simulink model "main"  (R2016b)
settings: Solver=FixedStepAuto  StartTime=0.0  StopTime=inf  FixedStep=Ts  MaxStep=0.2  RelTol=1e-2
undefined symbols (not defined in the file): checks, datetime, decyear, delta_e, deltae_degrees, deltafl_degrees, deltafr_degrees, deltar_degrees, deltat_1, deltat_2, deltat_3, deltat_4, deltat_5, Earth, F, ft, groundReaction, initialValues, juliandate, LD, leapyear, Light, m, MIL, Newton, Raphson, s, sigbuilder_block, Ts, WGS84
libraries: simulink x68, aerolibutil x17, aerolibtransform2 x15, simulink_extras x13, aerolibasang x5, aerolib6dofsys x5, aerolib6dof2 x4, aerolibwind2 x3, aerolibbdyn x3, vrlib x3, aerolibconvert2 x3, aerolibactuator x2
(part 8 of 10)

== system main/LIBIS Plant/Propulsion/Variant_Motor_5 ==
  note: 1) Add Subsystem or Model blocks as valid variant choices.
      | 2) You cannot connect blocks at this level. At simulation, connectivity is automatically
      | determined, based on the active variant and port name matching.
  Vbattery : Inport
  Throttle : Inport  Port=2
  envData : Inport  Port=3
  plantData : Inport  Port=4
  mappedMotor_5 : Subsystem  VariantControl=mappedMotors==1
  noMappedMotor_5 : Subsystem  VariantControl=mappedMotors~=1
  Im : Outport
  Thrust : Outport  Port=2
  Thrust_moment : Outport  Port=3

== system main/LIBIS Plant/Subsystem/calc alpha_dot ==
  q : Inport
  alpha,beta : Inport  Port=2
  Ab : Inport  Port=3
  Vw : Inport  Port=4
  Direction Cosine Matrix Body to Wind : aerolibtransform2/Direction Cosine Matrix Body to Wind
  Product1 : Product  Multiplication=Matrix(*)  SaturateOnIntegerOverflow=on  InputSameDT=on  OutDataTypeStr=Inherit: Same as first input
  Product2 : Product  Inputs=*/  SaturateOnIntegerOverflow=on  InputSameDT=on  OutDataTypeStr=Inherit: Same as first input
  Selector2 : Selector  IndexMode=Zero-based  InputPortWidth=3  IndexOptions=Index vector (dialog)  Indices=2  OutputSizes=1
  Selector3 : Selector  IndexMode=Zero-based  InputPortWidth=3  IndexOptions=Index vector (dialog)  Indices=0  OutputSizes=1
  Sum : Sum  Inputs=++|
  Transpose1 : Math  Operator=transpose  SaturateOnIntegerOverflow=on
  alpha_dot : Outport
  wires:
  Direction Cosine Matrix Body to Wind/1 -> Transpose1/1
  Transpose1/1 -> Product1/1
  Product1/1 -> Selector2/1
  Selector2/1 -> Product2/1
  Selector3/1 -> Product2/2
  Product2/1 -> Sum/2
  alpha,beta/1 -> Direction Cosine Matrix Body to Wind/1
  q/1 -> Sum/1
  Sum/1 -> alpha_dot/1
  Ab/1 -> Product1/2
  Vw/1 -> Selector3/1

== system main/LIBIS Plant/alpha_dot, beta_dot/Subsystem ==
  beta : Inport  Unit=rad
  alpha : Inport  Port=2  Unit=rad
  V_body : Inport  Port=3  Unit=meter/s
  Omega_body : Inport  Port=4  Unit=rad/s
  Accel_body : Inport  Port=5  Unit=m/s^2
  Constant11 : Constant  Value=0
  Direction Cosine Matrix Body to Wind : aerolibtransform2/Direction Cosine Matrix Body to Wind
  Mux4 : Mux  Inputs=2
  Product1 : Product  Multiplication=Matrix(*)  SaturateOnIntegerOverflow=on  InputSameDT=on  OutDataTypeStr=Inherit: Same as first input
  Selector : Selector  InputPortWidth=3  IndexOptions=Index vector (dialog)  Indices=[2]  OutputSizes=1
  calc alpha_dot : Subsystem
  alpha_dot : Outport  Unit=rad/s
  beta_dot : Outport  Port=2
  wires:
  Direction Cosine Matrix Body to Wind/1 -> Product1/1
  Product1/1 -> calc alpha_dot/4(Vw)
  Mux4/1 -> Direction Cosine Matrix Body to Wind/1, calc alpha_dot/2(alpha,beta)
  Constant11/1 -> beta_dot/1  "beta_dot"
  alpha/1 -> Mux4/1
  Omega_body/1 -> Selector/1
  V_body/1 -> Product1/2
  Accel_body/1 -> calc alpha_dot/3(Ab)
  beta/1 -> Mux4/2
  calc alpha_dot/1(alpha_dot) -> alpha_dot/1
  Selector/1 -> calc alpha_dot/1(q)  "q"

== system main/Sensors/Feedthrough Sensors/CPU ==
  States : Inport  OutDataTypeStr=Bus: plantDataBus
  Bus Selector : BusSelector  OutputSignals=CG,remainingCapacity
  CGMeas : Outport
  remainingCapacityMeas : Outport  Port=2
  wires:
  States/1 -> Bus Selector/1  "plantData"
  Bus Selector/1 -> CGMeas/1  "<CG>"
  Bus Selector/2 -> remainingCapacityMeas/1  "<remainingCapacity>"

== system main/Sensors/Feedthrough Sensors/GPS ==
  States : Inport  OutDataTypeStr=Bus: plantDataBus
  Bus Creator : BusCreator  Inputs='LatitudeMeas_deg','LongitudeMeas_deg','AltitudeMeas_m'  OutDataTypeStr=Bus: LLAMeasBus  NonVirtualBus=on
  Bus Selector : BusSelector  OutputSignals=LLA.Latitude_deg,LLA.Longitude_deg,LLA.Altitude_m
  Constant13 : Constant  Value=initialValues.href
  Derivative : Derivative
  LLA to Flat Earth : aerolibtransform2/LLA to Flat Earth  units=Metric (MKS)  ptype=Earth (WGS84)  F=1/298.257223563  R=6378137  LL0=initialValues.LatLong0  psi=0
  Mux2 : Mux  Inputs=2
  Signal Specification : SignalSpecification
  Signal Specification1 : SignalSpecification
  Signal Specification2 : SignalSpecification
  LLAMeas : Outport  OutDataTypeStr=Bus: LLAMeasBus
  X_nedMeas : Outport  Port=2
  VearthMeas : Outport  Port=3
  wires:
  Bus Creator/1 -> LLAMeas/1  "LLAMeas"
  Bus Selector/1 -> Signal Specification/1  "<Latitude_deg>"
  Bus Selector/3 -> Signal Specification2/1  "<Altitude_m>"
  Bus Selector/2 -> Signal Specification1/1  "<Longitude_deg>"
  Signal Specification/1 -> Mux2/1, Bus Creator/1  "LatitudeMeas_deg"
  Signal Specification1/1 -> Mux2/2, Bus Creator/2  "LongitudeMeas_deg"
  Signal Specification2/1 -> LLA to Flat Earth/2, Bus Creator/3  "AltitudeMeas_m"
  States/1 -> Bus Selector/1  "plantData"
  Constant13/1 -> LLA to Flat Earth/3
  Mux2/1 -> LLA to Flat Earth/1
  LLA to Flat Earth/1 -> Derivative/1, X_nedMeas/1  "X_NedMeas"
  Derivative/1 -> VearthMeas/1

== system main/Sensors/Feedthrough Sensors/IMU ==
  States : Inport  OutDataTypeStr=Bus: plantDataBus
  Environment : Inport  Port=2  OutDataTypeStr=Bus: envDataBus
  Bus Creator : BusCreator  Inputs='pMeas','qMeas','rMeas'  OutDataTypeStr=Bus: OmegaMeasBus  NonVirtualBus=on
  Bus Selector : BusSelector  OutputSignals=Accel_body,Omega_body.p,Omega_body.q,Omega_body.r,dOmega_body,CG,DCM_body_earth
  Bus Selector1 : BusSelector  OutputSignals=Gravity_ned
  Calculate DCM & Euler Angles : Subsystem
  Demux : Demux  Outputs=3
  Mux : Mux  Inputs=3
  Mux1 : Mux  Inputs=3
  Product : Product  Multiplication=Matrix(*)
  Three-axis Inertial Measurement Unit : aerolibnav/Three-axis Inertial Measurement Unit  units=Metric (MKS)  imu=[0 0 0]  i_Ts=0  dtype_a=off  w_a=190  z_a=1  a_sf_cc=[1 0 0; 0 1 0; 0 0 1]  a_bias=[0 0 0]  a_sat="[-inf  -inf  -inf  inf inf inf]"  dtype_g=off  w_g=190  z_g=1  g_sf_cc=[1 0 0; 0 1 0; 0 0 1]  g_bias=[0 0 0]  g_sens=[0 0 0]  g_sat="[-inf  -inf  -inf  inf inf inf]"  i_rand=off  i_seeds=[23093 23094 23095 23096 23097 23098]  i_pow=[0.001 0.001 0.001 0.0001 0.0001 0.0001]
  AccelMeas_body : Outport
  OmegaMeas_body : Outport  Port=2  OutDataTypeStr=Bus: OmegaMeasBus
  DCMMeas_body_earth : Outport  Port=3
  EulerMeas : Outport  Port=4
  wires:
  Demux/1 -> Mux/1, Bus Creator/1  "pMeas"
  Demux/2 -> Mux/2, Bus Creator/2  "qMeas"
  Demux/3 -> Mux/3, Bus Creator/3  "rMeas"
  Calculate DCM & Euler Angles/1(DCMMeas) -> DCMMeas_body_earth/1
  Calculate DCM & Euler Angles/2(EulerMeas) -> EulerMeas/1
  Mux/1 -> Calculate DCM & Euler Angles/1("p q r ")
  Three-axis Inertial Measurement Unit/1 -> AccelMeas_body/1
  Bus Creator/1 -> OmegaMeas_body/1
  Three-axis Inertial Measurement Unit/2 -> Demux/1
  States/1 -> Bus Selector/1  "plantData"
  Bus Selector/4 -> Mux1/3  "<r>"
  Bus Selector/3 -> Mux1/2  "<q>"
  Bus Selector/2 -> Mux1/1  "<p>"
  Environment/1 -> Bus Selector1/1  "Environment"
  Bus Selector1/1 -> Product/2  "<Gravity_ned>"
  Mux1/1 -> Three-axis Inertial Measurement Unit/2  "Omega_body"
  Bus Selector/1 -> Three-axis Inertial Measurement Unit/1  "<Accel_body>"
  Bus Selector/6 -> Three-axis Inertial Measurement Unit/4  "<CG>"
  Bus Selector/5 -> Three-axis Inertial Measurement Unit/3  "<dOmega_body>"
  Bus Selector/7 -> Product/1  "<DCM_body_earth>"
  Product/1 -> Three-axis Inertial Measurement Unit/5

== system main/Sensors/Feedthrough Sensors/Pitot ==
  States : Inport  OutDataTypeStr=Bus: plantDataBus
  Environment : Inport  Port=2  OutDataTypeStr=Bus: envDataBus
  Bus Selector : BusSelector  OutputSignals=V_body
  Bus Selector1 : BusSelector  OutputSignals=windVelocity
  Sum : Sum  Inputs=|+-
  VaeroMeas_body : Outport
  wires:
  Bus Selector/1 -> Sum/1  "<V_body>"
  States/1 -> Bus Selector/1  "plantData"
  Environment/1 -> Bus Selector1/1
  Bus Selector1/1 -> Sum/2  "<windVelocity>"
  Sum/1 -> VaeroMeas_body/1  "VaeroMeas_body"

== system main/Sensors/Feedthrough Sensors/Veleta ==
  States : Inport  OutDataTypeStr=Bus: plantDataBus
  Bus Selector : BusSelector  OutputSignals=alpha,beta
  alphaMeas : Outport
  betaMeas : Outport  Port=2
  wires:
  States/1 -> Bus Selector/1  "plantData"
  Bus Selector/1 -> alphaMeas/1  "<alpha>"
  Bus Selector/2 -> betaMeas/1  "<beta>"

== system main/Sensors/Noisy Sensors/CPU (Feedthough) ==
  States : Inport  OutDataTypeStr=Bus: plantDataBus
  Bus Selector : BusSelector  OutputSignals=CG,remainingCapacity
  CGMeas : Outport
  remainingCapacityMeas : Outport  Port=2
  wires:
  States/1 -> Bus Selector/1  "plantData"
  Bus Selector/1 -> CGMeas/1  "<CG>"
  Bus Selector/2 -> remainingCapacityMeas/1  "<remainingCapacity>"

== system main/Sensors/Noisy Sensors/GPS (Feedthough) ==
  States : Inport  OutDataTypeStr=Bus: plantDataBus
  Bus Creator : BusCreator  Inputs='LatitudeMeas_deg','LongitudeMeas_deg','AltitudeMeas_m'  OutDataTypeStr=Bus: LLAMeasBus  NonVirtualBus=on
  Bus Selector : BusSelector  OutputSignals=LLA.Latitude_deg,LLA.Longitude_deg,LLA.Altitude_m
  Constant13 : Constant  Value=initialValues.href
  Derivative : Derivative
  LLA to Flat Earth : aerolibtransform2/LLA to Flat Earth  units=Metric (MKS)  ptype=Earth (WGS84)  F=1/298.257223563  R=6378137  LL0=initialValues.LatLong0  psi=0
  Mux2 : Mux  Inputs=2
  Signal Specification : SignalSpecification
  Signal Specification1 : SignalSpecification
  Signal Specification2 : SignalSpecification
  LLAMeas : Outport  OutDataTypeStr=Bus: LLAMeasBus
  X_nedMeas : Outport  Port=2
  VearthMeas : Outport  Port=3
  wires:
  Bus Creator/1 -> LLAMeas/1  "LLAMeas"
  Bus Selector/1 -> Signal Specification/1  "<Latitude_deg>"
  Bus Selector/3 -> Signal Specification2/1  "<Altitude_m>"
  Bus Selector/2 -> Signal Specification1/1  "<Longitude_deg>"
  Signal Specification/1 -> Mux2/1, Bus Creator/1  "LatitudeMeas_deg"
  Signal Specification1/1 -> Mux2/2, Bus Creator/2  "LongitudeMeas_deg"
  Signal Specification2/1 -> LLA to Flat Earth/2, Bus Creator/3  "AltitudeMeas_m"
  States/1 -> Bus Selector/1  "plantData"
  Constant13/1 -> LLA to Flat Earth/3
  Mux2/1 -> LLA to Flat Earth/1
  LLA to Flat Earth/1 -> Derivative/1, X_nedMeas/1  "X_NedMeas"
  Derivative/1 -> VearthMeas/1

== system main/Sensors/Noisy Sensors/IMU ==
  States : Inport  OutDataTypeStr=Bus: plantDataBus
  Environment : Inport  Port=2  OutDataTypeStr=Bus: envDataBus
  Bus Creator : BusCreator  Inputs='pMeas','qMeas','rMeas'  OutDataTypeStr=Bus: OmegaMeasBus  NonVirtualBus=on
  Bus Selector : BusSelector  OutputSignals=Accel_body,Omega_body.p,Omega_body.q,Omega_body.r,dOmega_body,CG,DCM_body_earth
  Bus Selector1 : BusSelector  OutputSignals=Gravity_ned
  Calculate DCM & Euler Angles : Subsystem
  Demux : Demux  Outputs=3
  Mux : Mux  Inputs=3
  Mux1 : Mux  Inputs=3
  Product : Product  Multiplication=Matrix(*)
  Three-axis Inertial Measurement Unit : aerolibnav/Three-axis Inertial Measurement Unit  units=Metric (MKS)  imu=[0 0 0]  i_Ts=0  dtype_a=on  w_a=190  z_a=0.707  a_sf_cc=[1 0 0; 0 1 0; 0 0 1]  a_bias=[0 0 0]  a_sat="[-inf  -inf  -inf  inf inf inf]"  dtype_g=on  w_g=190  z_g=0.707  g_sf_cc=[1 0 0; 0 1 0; 0 0 1]  g_bias=[0 0 0]  g_sens=[0 0 0]  g_sat="[-inf  -inf  -inf  inf inf inf]"  i_rand=on  i_seeds=[23093 23094 23095 23096 23097 23098]  i_pow=[0.001 0.001 0.001 0.0001 0.0001 0.0001]
  AccelMeas_body : Outport
  OmegaMeas_body : Outport  Port=2  OutDataTypeStr=Bus: OmegaMeasBus
  DCMMeas_body_earth : Outport  Port=3
  EulerMeas : Outport  Port=4
  wires:
  States/1 -> Bus Selector/1  "plantData"
  Demux/1 -> Mux/1, Bus Creator/1  "pMeas"
  Demux/2 -> Mux/2, Bus Creator/2  "qMeas"
  Demux/3 -> Mux/3, Bus Creator/3  "rMeas"
  Bus Selector/4 -> Mux1/3  "<r>"
  Bus Selector/3 -> Mux1/2  "<q>"
  Bus Selector/2 -> Mux1/1  "<p>"
  Calculate DCM & Euler Angles/1(DCMMeas) -> DCMMeas_body_earth/1
  Calculate DCM & Euler Angles/2(EulerMeas) -> EulerMeas/1
  Mux/1 -> Calculate DCM & Euler Angles/1("p q r ")
  Environment/1 -> Bus Selector1/1  "Environment"
  Bus Selector1/1 -> Product/2  "<Gravity_ned>"
  Three-axis Inertial Measurement Unit/1 -> AccelMeas_body/1
  Mux1/1 -> Three-axis Inertial Measurement Unit/2  "Omega_body"
  Bus Selector/1 -> Three-axis Inertial Measurement Unit/1  "<Accel_body>"
  Bus Selector/6 -> Three-axis Inertial Measurement Unit/4  "<CG>"
  Bus Selector/5 -> Three-axis Inertial Measurement Unit/3  "<dOmega_body>"
  Bus Creator/1 -> OmegaMeas_body/1
  Three-axis Inertial Measurement Unit/2 -> Demux/1
  Bus Selector/7 -> Product/1  "<DCM_body_earth>"
  Product/1 -> Three-axis Inertial Measurement Unit/5

== system main/Sensors/Noisy Sensors/Pitot (Feedthough) ==
  States : Inport  OutDataTypeStr=Bus: plantDataBus
  Environment : Inport  Port=2  OutDataTypeStr=Bus: envDataBus
  Bus Selector : BusSelector  OutputSignals=V_body
  Bus Selector1 : BusSelector  OutputSignals=windVelocity
  Sum : Sum  Inputs=|+-
  VaeroMeas_body : Outport
  wires:
  Bus Selector/1 -> Sum/1  "<V_body>"
  States/1 -> Bus Selector/1  "plantData"
  Environment/1 -> Bus Selector1/1
  Bus Selector1/1 -> Sum/2  "<windVelocity>"
  Sum/1 -> VaeroMeas_body/1  "VaeroMeas_body"

== system main/Sensors/Noisy Sensors/Veleta (Feedthough) ==
  States : Inport  OutDataTypeStr=Bus: plantDataBus
  Bus Selector : BusSelector  OutputSignals=alpha,beta
  alphaMeas : Outport
  betaMeas : Outport  Port=2
  wires:
  States/1 -> Bus Selector/1  "plantData"
  Bus Selector/1 -> alphaMeas/1  "<alpha>"
  Bus Selector/2 -> betaMeas/1  "<beta>"

== system main/Visualization/Subsystem/Flightpath Angle ==
  Ve : Inport
  Constant : Constant  Value=eps
  Sum2 : Sum  Inputs=+  SaturateOnIntegerOverflow=on  InputSameDT=on  OutDataTypeStr=Inherit: Same as first input
  Switch : Switch  Criteria=u2 > Threshold
  product : Product  SaturateOnIntegerOverflow=on  InputSameDT=on  OutDataTypeStr=Inherit: Same as first input
  product1 : Product  Inputs=/*  SaturateOnIntegerOverflow=on  InputSameDT=on  OutDataTypeStr=Inherit: Same as first input
  rad-->deg4 : Gain  Gain=-1  SaturateOnIntegerOverflow=on  OutDataTypeStr=Inherit: Same as input  ParamDataTypeStr=Inherit: Same as input
  tangent : Trigonometry  Operator=atan
  u,v : Selector  IndexMode=Zero-based  InputPortWidth=3  IndexOptions=Index vector (dialog)  Indices=[0 1]  OutputSizes=1
  v : Sqrt  SaturateOnIntegerOverflow=on
  w : Selector  IndexMode=Zero-based  InputPortWidth=3  IndexOptions=Index vector (dialog)  Indices=2  OutputSizes=1
  gamma : Outport
  wires:
  Ve/1 -> w/1, u,v/1
  product/1 -> Sum2/1
  Sum2/1 -> v/1
  product1/1 -> tangent/1
  u,v/1 -> product/2, product/1
  w/1 -> rad-->deg4/1
  v/1 -> Switch/2, product1/1
  rad-->deg4/1 -> product1/2
  tangent/1 -> Switch/1
  Constant/1 -> Switch/3
  Switch/1 -> gamma/1

== system main/FCS/Quadcopter/Quad actuator commands/Altitude ==
  Altitude cmd : Inport
  Bias : Bias  Bias=LD.FCS.Quadcopter.Throttle.bias
  dThrottle : Gain  Gain=LD.FCS.Quadcopter.Throttle.dThrottle
  T5 : Outport
  T3 : Outport  Port=2
  T4 : Outport  Port=3
  T2 : Outport  Port=4
  wires:
  Bias/1 -> T5/1, T4/1, T3/1, T2/1
  Altitude cmd/1 -> dThrottle/1
  dThrottle/1 -> Bias/1

== system main/FCS/Quadcopter/Quad actuator commands/Pitch ==
  Pitch Cmd : Inport
  Constant1 : Constant  Value=LD.Inertia.CG
  Constant2 : Constant  Value=LD.Inertia.CG
  Divide : Product  Inputs=*/
  Product : Product
  Product1 : Product
  Selector : Selector  InputPortWidth=3  IndexOptions=Index vector (dialog)  Indices=1  OutputSizes=1
  Selector1 : Selector  InputPortWidth=3  IndexOptions=Index vector (dialog)  Indices=1  OutputSizes=1
  Sum1 : Sum  Inputs=+-|
  Sum2 : Sum  Inputs=+-|
  dPitch : Gain  Gain=LD.FCS.Quadcopter.Pitch.dPitch
  "motor2 position " : Constant  Value=LD.Propulsion.motor2.Position
  motor2 position 1 : Constant  Value=LD.Propulsion.motor3.Position
  T5 : Outport
  T3 : Outport  Port=2
  T2 : Outport  Port=3
  T4 : Outport  Port=4
  wires:
  Pitch Cmd/1 -> dPitch/1
  Product/1 -> T3/1
  dPitch/1 -> T5/1, Product1/1, Product/1, T2/1
  Constant1/1 -> Sum1/2
  "motor2 position "/1 -> Sum1/1
  Sum1/1 -> Selector/1  "arm"
  Constant2/1 -> Sum2/2
  motor2 position 1/1 -> Sum2/1
  Sum2/1 -> Selector1/1  "arm"
  Selector/1 -> Divide/1
  Selector1/1 -> Divide/2
  Product1/1 -> T4/1
  [Gain] -> Product/2
  [Gain] -> Product1/2
  Divide/1 -> [Gain]

== system main/FCS/Quadcopter/Quad actuator commands/Roll ==
  Roll Cmd : Inport
  Gain : Gain  Gain=-1
  Gain1 : Gain  Gain=-1
  dRoll : Gain  Gain=LD.FCS.Quadcopter.Roll.dRoll
  T4 : Outport
  T2 : Outport  Port=2
  T5 : Outport  Port=3
  T3 : Outport  Port=4
  wires:
  Gain/1 -> T2/1
  dRoll/1 -> Gain1/1, Gain/1, T4/1, T5/1
  Roll Cmd/1 -> dRoll/1
  Gain1/1 -> T3/1

== system main/FCS/Quadcopter/Quad actuator commands/Yaw ==
  Yaw Cmd : Inport
  Gain : Gain  Gain=-1
  Gain1 : Gain  Gain=-1
  dYaw : Gain  Gain=LD.FCS.Quadcopter.Yaw.dYaw
  T5 : Outport
  T4 : Outport  Port=2
  T3 : Outport  Port=3
  T2 : Outport  Port=4
  wires:
  Yaw Cmd/1 -> dYaw/1
  dYaw/1 -> Gain1/1, T4/1, T2/1, Gain/1
  Gain1/1 -> T5/1
  Gain/1 -> T3/1

== system main/FCS/Quadcopter --> Fixed-Wing/Quad actuator commands/Altitude ==
  Altitude cmd : Inport
  Bias : Bias  Bias=LD.FCS.Quadcopter.Throttle.bias
  dThrottle : Gain  Gain=LD.FCS.Quadcopter.Throttle.dThrottle
  T5 : Outport
  T3 : Outport  Port=2
  T4 : Outport  Port=3
  T2 : Outport  Port=4
  wires:
  Bias/1 -> T5/1, T4/1, T3/1, T2/1
  Altitude cmd/1 -> dThrottle/1
  dThrottle/1 -> Bias/1

== system main/FCS/Quadcopter --> Fixed-Wing/Quad actuator commands/Pitch ==
  Pitch Cmd : Inport
  Constant1 : Constant  Value=LD.Inertia.CG
  Constant2 : Constant  Value=LD.Inertia.CG
  Divide : Product  Inputs=*/
  Product : Product
  Product1 : Product
  Selector : Selector  InputPortWidth=3  IndexOptions=Index vector (dialog)  Indices=1  OutputSizes=1
  Selector1 : Selector  InputPortWidth=3  IndexOptions=Index vector (dialog)  Indices=1  OutputSizes=1
  Sum1 : Sum  Inputs=+-|
  Sum2 : Sum  Inputs=+-|
  dPitch : Gain  Gain=LD.FCS.Quadcopter.Pitch.dPitch
  "motor2 position " : Constant  Value=LD.Propulsion.motor2.Position
  motor2 position 1 : Constant  Value=LD.Propulsion.motor3.Position
  T5 : Outport
  T3 : Outport  Port=2
  T2 : Outport  Port=3
  T4 : Outport  Port=4
  wires:
  Pitch Cmd/1 -> dPitch/1
  Product/1 -> T3/1
  dPitch/1 -> T5/1, Product1/1, Product/1, T2/1
  Constant1/1 -> Sum1/2
  "motor2 position "/1 -> Sum1/1
  Sum1/1 -> Selector/1  "arm"
  Constant2/1 -> Sum2/2
  motor2 position 1/1 -> Sum2/1
  Sum2/1 -> Selector1/1  "arm"
  Selector/1 -> Divide/1
  Selector1/1 -> Divide/2
  Product1/1 -> T4/1
  [Gain] -> Product/2
  [Gain] -> Product1/2
  Divide/1 -> [Gain]

== system main/FCS/Quadcopter --> Fixed-Wing/Quad actuator commands/Roll ==
  Roll Cmd : Inport
  Gain : Gain  Gain=-1
  Gain1 : Gain  Gain=-1
  dRoll : Gain  Gain=LD.FCS.Quadcopter.Roll.dRoll
  T4 : Outport
  T2 : Outport  Port=2
  T5 : Outport  Port=3
  T3 : Outport  Port=4
  wires:
  Gain/1 -> T2/1
  dRoll/1 -> Gain1/1, Gain/1, T4/1, T5/1
  Roll Cmd/1 -> dRoll/1
  Gain1/1 -> T3/1

== system main/FCS/Quadcopter --> Fixed-Wing/Quad actuator commands/Yaw ==
  Yaw Cmd : Inport
  Gain : Gain  Gain=-1
  Gain1 : Gain  Gain=-1
  dYaw : Gain  Gain=LD.FCS.Quadcopter.Yaw.dYaw
  T5 : Outport
  T4 : Outport  Port=2
  T3 : Outport  Port=3
  T2 : Outport  Port=4
  wires:
  Yaw Cmd/1 -> dYaw/1
  dYaw/1 -> Gain1/1, T4/1, T2/1, Gain/1
  Gain1/1 -> T5/1
  Gain/1 -> T3/1

== system main/LIBIS Plant/Propulsion/Variant_Motor_1/mappedMotor_1 ==
  Vbattery : Inport
  Throttle : Inport  Port=2
  envData : Inport  Port=3
  plantData : Inport  Port=4
  3x3 Cross Product : aerolibutil/3x3 Cross Product
  Bus Selector : BusSelector  OutputSignals=V_body,CG,LLA.Altitude_m
  Bus Selector1 : BusSelector  OutputSignals=windVelocity
  Constant{1..4} (4 alike) : Constant  Value=0
  ESC_1 : Subsystem
  Motor and Propeller Coupling_1 : Subsystem
  Mux : Mux  Inputs=3
  Mux1 : Mux  Inputs=3
  Selector1 : Selector  InputPortWidth=3  IndexOptions=Index vector (dialog)  Indices=[1]  OutputSizes=1
  Selector2 : Selector  InputPortWidth=3  IndexOptions=Index vector (dialog)  Indices=[1]  OutputSizes=1
  Sum : Sum  Inputs=|+-
  Sum1 : Sum  Inputs=+-|
  Sum2 : Sum  Inputs=|++
  Terminator : Terminator
  Torque : Subsystem
  "motor2 position " : Constant  Value=LD.Propulsion.motor1.Position
  Im : Outport
  Thrust : Outport  Port=2
  Thrust_moment : Outport  Port=3
  wires:
  Vbattery/1 -> ESC_1/1(V_battery)
  ESC_1/1(V_ESC) -> Motor and Propeller Coupling_1/1(Voltage)  "V_ESC"
  Mux/1 -> Thrust/1, 3x3 Cross Product/2  "Thrust_vector"
  Throttle/1 -> ESC_1/2(Throttle)
  Constant1/1 -> Mux/2
  Sum1/1 -> 3x3 Cross Product/1  "arm"
  Motor and Propeller Coupling_1/3(Current) -> Im/1
  Bus Selector/2 -> [CG]  "<CG>"
  Bus Selector/3 -> [Altitude]  "<Altitude_m>"
  Bus Selector1/1 -> [V_wind]  "<windVelocity>"
  [CG] -> Sum1/2
  Selector2/1 -> Sum/1
  Selector1/1 -> Sum/2
  plantData/1 -> Bus Selector/1
  [V_body] -> Selector2/1
  Motor and Propeller Coupling_1/1(Thrust) -> Mux/1  "Thrust_scalar"
  [Altitude] -> Motor and Propeller Coupling_1/2(Height)
  "motor2 position "/1 -> Sum1/1
  [V_wind] -> Selector1/1
  Constant2/1 -> Mux/3
  Bus Selector/1 -> [V_body]  "<V_body>"
  envData/1 -> Bus Selector1/1
  Motor and Propeller Coupling_1/2(Power) -> Terminator/1
  Sum/1 -> Torque/2(Vflight), Motor and Propeller Coupling_1/3(Vflight)
  Mux1/1 -> Sum2/2  "Torque_vector"
  Constant3/1 -> Mux1/2
  Sum2/1 -> Thrust_moment/1
  3x3 Cross Product/1 -> Sum2/1
  Motor and Propeller Coupling_1/4(RPM) -> Torque/1(RPM)  "RPM"
  Constant4/1 -> Mux1/3
  Torque/1(Torque) -> Mux1/1

== system main/LIBIS Plant/Propulsion/Variant_Motor_1/noMappedMotor_1 ==
  Vbattery : Inport
  Throttle : Inport  Port=2
  envData : Inport  Port=3
  plantData : Inport  Port=4
  3x3 Cross Product : aerolibutil/3x3 Cross Product
  Algebraic Constraint : simulink/Math Operations/Algebraic Constraint  z0=0
  Bus Selector : BusSelector  OutputSignals=V_body,CG
  Bus Selector1 : BusSelector  OutputSignals=windVelocity,AirDensity
  Constant{1..4} (4 alike) : Constant  Value=0
  ESC_1 : Subsystem
  Motor_1 : Subsystem
  Mux : Mux  Inputs=3
  Mux1 : Mux  Inputs=3
  Propeller_1 : Subsystem
  Selector1 : Selector  InputPortWidth=3  IndexOptions=Index vector (dialog)  Indices=[1]  OutputSizes=1
  Selector3 : Selector  InputPortWidth=3  IndexOptions=Index vector (dialog)  Indices=[1]  OutputSizes=1
  Sum : Sum  Inputs=|+-
  Sum1 : Sum  Inputs=+|-
  Sum2 : Sum  Inputs=|+-
  Sum3 : Sum  Inputs=++|
  Torque : Subsystem
  "motor1 position " : Constant  Value=LD.Propulsion.motor1.Position
  Im : Outport
  Thrust : Outport  Port=2
  Thrust_moment : Outport  Port=3
  wires:
  Throttle/1 -> ESC_1/2(Throttle)
  Vbattery/1 -> ESC_1/1(V_battery)
  Motor_1/2(Peje) -> Sum/1  "P_available"
  Motor_1/1(RPM) -> Torque/1(RPM), Propeller_1/1(RPM)  "RPM"
  "motor1 position "/1 -> Sum1/1
  Sum/1 -> Algebraic Constraint/1  "P_error"
  Algebraic Constraint/1 -> Im/1, Motor_1/2(Im)  "Im"
  Sum1/1 -> 3x3 Cross Product/1  "arm"
  Propeller_1/1(P_needed) -> Sum/2  "P_needed"
  Mux/1 -> Thrust/1, 3x3 Cross Product/2  "Thrust_vector1"
  Propeller_1/2(Thrust) -> Mux/1  "Thrust_scalar"
  Constant1/1 -> Mux/2
  Constant2/1 -> Mux/3
  [CG] -> Sum1/2
  ESC_1/1(V_ESC) -> Motor_1/1(V_ESC)
  plantData/1 -> Bus Selector/1
  Bus Selector/1 -> [V_body]  "<V_body>"
  Bus Selector/2 -> [CG]  "<CG>"
  [V_body] -> Selector3/1
  [V_wind] -> Selector1/1
  Selector1/1 -> Sum2/2
  Selector3/1 -> Sum2/1
  envData/1 -> Bus Selector1/1
  Bus Selector1/1 -> [V_wind]  "<windVelocity>"
  Bus Selector1/2 -> [AirDensity]  "<AirDensity>"
  [AirDensity] -> Propeller_1/3(airDensity)
  Constant3/1 -> Mux1/2
  Constant4/1 -> Mux1/3
  Torque/1(Torque) -> Mux1/1
  Mux1/1 -> Sum3/1  "Torque_vector"
  Sum3/1 -> Thrust_moment/1
  3x3 Cross Product/1 -> Sum3/2
  Sum2/1 -> Propeller_1/2(V_flight), Torque/2(Vflight)

== system main/LIBIS Plant/Propulsion/Variant_Motor_2/mappedMotor_2 ==
  Vbattery : Inport
  Throttle : Inport  Port=2
  envData : Inport  Port=3
  plantData : Inport  Port=4
  3x3 Cross Product : aerolibutil/3x3 Cross Product
  Bus Selector : BusSelector  OutputSignals=V_body,CG,LLA.Altitude_m
  Bus Selector1 : BusSelector  OutputSignals=windVelocity
  Constant{1..4} (4 alike) : Constant  Value=0
  ESC_2 : Subsystem
  Motor and Propeller Coupling_2 : Subsystem
  Mux : Mux  Inputs=3
  Mux1 : Mux  Inputs=3
  Selector1 : Selector  InputPortWidth=3  IndexOptions=Index vector (dialog)  Indices=[3]  OutputSizes=1
  Selector2 : Selector  InputPortWidth=3  IndexOptions=Index vector (dialog)  Indices=[3]  OutputSizes=1
  Sum : Sum  Inputs=|+-
  Sum1 : Sum  Inputs=+-|
  Sum2 : Sum  Inputs=|++
  Terminator : Terminator
  Torque : Subsystem
  Unary Minus : UnaryMinus
  "motor2 position " : Constant  Value=LD.Propulsion.motor2.Position
  Im : Outport
  Thrust : Outport  Port=2
  Thrust_moment : Outport  Port=3
  wires:
  ESC_2/1(V_ESC) -> Motor and Propeller Coupling_2/1(Voltage)  "V_ESC"
  [V_body] -> Selector2/1
  Vbattery/1 -> ESC_2/1(V_battery)
  Bus Selector/1 -> [V_body]  "<V_body>"
  Motor and Propeller Coupling_2/1(Thrust) -> Unary Minus/1  "Thrust_scalar"
  Unary Minus/1 -> Mux/3
  Bus Selector/3 -> [Altitude]  "<Altitude_m>"
  [CG] -> Sum1/2
  "motor2 position "/1 -> Sum1/1
  Motor and Propeller Coupling_2/3(Current) -> Im/1
  Sum1/1 -> 3x3 Cross Product/1  "arm"
  Constant2/1 -> Mux/1
  Mux/1 -> Thrust/1, 3x3 Cross Product/2  "Thrust_vector"
  Constant1/1 -> Mux/2
  Throttle/1 -> ESC_2/2(Throttle)
  plantData/1 -> Bus Selector/1
  Bus Selector/2 -> [CG]  "<CG>"
  [V_wind] -> Selector1/1
  [Altitude] -> Motor and Propeller Coupling_2/2(Height)
  Sum/1 -> Torque/2(Vflight), Motor and Propeller Coupling_2/3(Vflight)
  Motor and Propeller Coupling_2/4(RPM) -> Torque/1(RPM)
  Motor and Propeller Coupling_2/2(Power) -> Terminator/1
  envData/1 -> Bus Selector1/1
  Selector1/1 -> Sum/2
  Bus Selector1/1 -> [V_wind]  "<windVelocity>"
  Selector2/1 -> Sum/1
  Constant4/1 -> Mux1/1
  Mux1/1 -> Sum2/2  "Torque_vector"
  Constant3/1 -> Mux1/2
  Sum2/1 -> Thrust_moment/1
  3x3 Cross Product/1 -> Sum2/1
  Torque/1(Torque) -> Mux1/3  "Torque"

== system main/LIBIS Plant/Propulsion/Variant_Motor_2/noMappedMotor_2 ==
  Vbattery : Inport
  Throttle : Inport  Port=2
  envData : Inport  Port=3
  plantData : Inport  Port=4
  3x3 Cross Product : aerolibutil/3x3 Cross Product
  Algebraic Constraint : simulink/Math Operations/Algebraic Constraint  z0=0
  Bus Selector : BusSelector  OutputSignals=V_body,CG
  Bus Selector1 : BusSelector  OutputSignals=windVelocity,AirDensity
  Constant{1..4} (4 alike) : Constant  Value=0
  ESC_2 : Subsystem
  Motor_2 : Subsystem
  Mux : Mux  Inputs=3
  Mux1 : Mux  Inputs=3
  Propeller_2 : Subsystem
  Selector1 : Selector  InputPortWidth=3  IndexOptions=Index vector (dialog)  Indices=[3]  OutputSizes=1
  Selector3 : Selector  InputPortWidth=3  IndexOptions=Index vector (dialog)  Indices=[3]  OutputSizes=1
  Sum : Sum  Inputs=|+-
  Sum1 : Sum  Inputs=+|-
  Sum2 : Sum  Inputs=|+-
  Sum3 : Sum  Inputs=++|
  Torque : Subsystem
  Unary Minus : UnaryMinus
  "motor2 position " : Constant  Value=LD.Propulsion.motor2.Position
  Im : Outport
  Thrust : Outport  Port=2
  Thrust_moment : Outport  Port=3
  wires:
  [AirDensity] -> Propeller_2/3(airDensity)
  Sum1/1 -> 3x3 Cross Product/1  "arm"
  Throttle/1 -> ESC_2/2(Throttle)
  Mux/1 -> Thrust/1, 3x3 Cross Product/2  "Thrust_vector1"
  Sum/1 -> Algebraic Constraint/1  "P_error"
  Propeller_2/1(P_needed) -> Sum/2  "P_needed"
  Vbattery/1 -> ESC_2/1(V_battery)
  Motor_2/1(RPM) -> Torque/1(RPM), Propeller_2/1(RPM)  "RPM"
  [CG] -> Sum1/2
  Constant2/1 -> Mux/1
  plantData/1 -> Bus Selector/1
  Motor_2/2(Peje) -> Sum/1  "P_available"
  Bus Selector/1 -> [V_body]  "<V_body>"
  Constant1/1 -> Mux/2
  Bus Selector/2 -> [CG]  "<CG>"
  "motor2 position "/1 -> Sum1/1
  ESC_2/1(V_ESC) -> Motor_2/1(V_ESC)  "V_ESC"
  Algebraic Constraint/1 -> Im/1, Motor_2/2(Im)  "Im"
  Propeller_2/2(Thrust) -> Unary Minus/1  "Thrust_scalar"
  Unary Minus/1 -> Mux/3
  [V_body] -> Selector3/1
  [V_wind] -> Selector1/1
  Sum2/1 -> Torque/2(Vflight), Propeller_2/2(V_flight)
  Selector1/1 -> Sum2/2
  Selector3/1 -> Sum2/1
  envData/1 -> Bus Selector1/1
  Bus Selector1/1 -> [V_wind]  "<windVelocity>"
  Bus Selector1/2 -> [AirDensity]  "<AirDensity>"
  Constant4/1 -> Mux1/1
  Constant3/1 -> Mux1/2
  Torque/1(Torque) -> Mux1/3  "Torque"
  3x3 Cross Product/1 -> Sum3/2
  Sum3/1 -> Thrust_moment/1
  Mux1/1 -> Sum3/1  "Torque_vector"

== system main/LIBIS Plant/Propulsion/Variant_Motor_3/mappedMotor_3 ==
  Vbattery : Inport
  Throttle : Inport  Port=2
  envData : Inport  Port=3
  plantData : Inport  Port=4
  3x3 Cross Product : aerolibutil/3x3 Cross Product
  Bus Selector : BusSelector  OutputSignals=V_body,CG,LLA.Altitude_m
  Bus Selector1 : BusSelector  OutputSignals=windVelocity
  Constant{1..4} (4 alike) : Constant  Value=0
  ESC_3 : Subsystem
  Motor and Propeller Coupling_3 : Subsystem
  Mux : Mux  Inputs=3
  Mux1 : Mux  Inputs=3
  Selector1 : Selector  InputPortWidth=3  IndexOptions=Index vector (dialog)  Indices=[3]  OutputSizes=1
  Selector2 : Selector  InputPortWidth=3  IndexOptions=Index vector (dialog)  Indices=[3]  OutputSizes=1
  Sum : Sum  Inputs=|+-
  Sum1 : Sum  Inputs=+-|
  Sum2 : Sum  Inputs=|++
  Terminator : Terminator
  Torque : Subsystem
  Unary Minus : UnaryMinus
  Unary Minus1 : UnaryMinus
  "motor2 position " : Constant  Value=LD.Propulsion.motor3.Position
  Im : Outport
  Thrust : Outport  Port=2
  Thrust_moment : Outport  Port=3
  wires:
  ESC_3/1(V_ESC) -> Motor and Propeller Coupling_3/1(Voltage)  "V_ESC"
  [V_wind] -> Selector1/1
  Motor and Propeller Coupling_3/1(Thrust) -> Unary Minus/1  "Thrust_scalar"
  Motor and Propeller Coupling_3/2(Power) -> Terminator/1
  Throttle/1 -> ESC_3/2(Throttle)
  Selector2/1 -> Sum/1
  Selector1/1 -> Sum/2
  Mux/1 -> Thrust/1, 3x3 Cross Product/2  "Thrust_vector"
  Motor and Propeller Coupling_3/3(Current) -> Im/1
  [V_body] -> Selector2/1
  plantData/1 -> Bus Selector/1
  Constant1/1 -> Mux/2
  envData/1 -> Bus Selector1/1
  Sum1/1 -> 3x3 Cross Product/1  "arm"
  Bus Selector/1 -> [V_body]  "<V_body>"
  Bus Selector/2 -> [CG]  "<CG>"
  Constant2/1 -> Mux/1
  Unary Minus/1 -> Mux/3
  [Altitude] -> Motor and Propeller Coupling_3/2(Height)
  "motor2 position "/1 -> Sum1/1
  Bus Selector1/1 -> [V_wind]  "<windVelocity>"
  [CG] -> Sum1/2
  Vbattery/1 -> ESC_3/1(V_battery)
  Bus Selector/3 -> [Altitude]  "<Altitude_m>"
  Sum/1 -> Torque/2(Vflight), Motor and Propeller Coupling_3/3(Vflight)
  Motor and Propeller Coupling_3/4(RPM) -> Torque/1(RPM)  "RPM"
  Constant4/1 -> Mux1/1
  Mux1/1 -> Sum2/2  "Torque_vector"
  Constant3/1 -> Mux1/2
  Sum2/1 -> Thrust_moment/1
  3x3 Cross Product/1 -> Sum2/1
  Torque/1(Torque) -> Unary Minus1/1
  Unary Minus1/1 -> Mux1/3

== system main/LIBIS Plant/Propulsion/Variant_Motor_3/noMappedMotor_3 ==
  Vbattery : Inport
  Throttle : Inport  Port=2
  envData : Inport  Port=3
  plantData : Inport  Port=4
  3x3 Cross Product : aerolibutil/3x3 Cross Product
  Algebraic Constraint : simulink/Math Operations/Algebraic Constraint  z0=0
  Bus Selector : BusSelector  OutputSignals=V_body,CG
  Bus Selector1 : BusSelector  OutputSignals=windVelocity,AirDensity
  Constant{1..4} (4 alike) : Constant  Value=0
  ESC_3 : Subsystem
  Motor_3 : Subsystem
  Mux : Mux  Inputs=3
  Mux1 : Mux  Inputs=3
  Propeller_3 : Subsystem
  Selector1 : Selector  InputPortWidth=3  IndexOptions=Index vector (dialog)  Indices=[3]  OutputSizes=1
  Selector3 : Selector  InputPortWidth=3  IndexOptions=Index vector (dialog)  Indices=[3]  OutputSizes=1
  Sum : Sum  Inputs=|+-
  Sum1 : Sum  Inputs=+|-
  Sum2 : Sum  Inputs=|+-
  Sum3 : Sum  Inputs=++|
  Torque : Subsystem
  Unary Minus : UnaryMinus
  Unary Minus1 : UnaryMinus
  "motor3 position " : Constant  Value=LD.Propulsion.motor3.Position
  Im : Outport
  Thrust : Outport  Port=2
  Thrust_moment : Outport  Port=3
  wires:
  Throttle/1 -> ESC_3/2(Throttle)
  Vbattery/1 -> ESC_3/1(V_battery)
  Propeller_3/2(Thrust) -> Unary Minus/1  "Thrust_scalar"
  Motor_3/2(Peje) -> Sum/1  "P_available"
  Sum1/1 -> 3x3 Cross Product/1  "arm"
  "motor3 position "/1 -> Sum1/1
  Mux/1 -> Thrust/1, 3x3 Cross Product/2  "Thrust_vector1"
  Constant1/1 -> Mux/2
  Constant2/1 -> Mux/1
  Algebraic Constraint/1 -> Im/1, Motor_3/2(Im)  "Im"
  [CG] -> Sum1/2
  ESC_3/1(V_ESC) -> Motor_3/1(V_ESC)
  Sum/1 -> Algebraic Constraint/1  "P_error"
  Unary Minus/1 -> Mux/3
  Propeller_3/1(P_needed) -> Sum/2  "P_needed"
  plantData/1 -> Bus Selector/1
  Bus Selector/1 -> [V_body]  "<V_body>"
  Bus Selector/2 -> [CG]  "<CG>"
  envData/1 -> Bus Selector1/1
  Bus Selector1/1 -> [V_wind]  "<windVelocity>"
  Bus Selector1/2 -> [AirDensity]  "<AirDensity>"
  [V_body] -> Selector3/1
  [V_wind] -> Selector1/1
  Selector1/1 -> Sum2/2
  Selector3/1 -> Sum2/1
  [AirDensity] -> Propeller_3/3(airDensity)
  Motor_3/1(RPM) -> Torque/1(RPM), Propeller_3/1(RPM)  "RPM"
  Sum2/1 -> Torque/2(Vflight), Propeller_3/2(V_flight)
  Constant4/1 -> Mux1/1
  Constant3/1 -> Mux1/2
  Torque/1(Torque) -> Mux1/3  "Torque"
  Sum3/1 -> Thrust_moment/1
  3x3 Cross Product/1 -> Sum3/2
  Unary Minus1/1 -> Sum3/1
  Mux1/1 -> Unary Minus1/1  "Torque_vector"

== system main/LIBIS Plant/Propulsion/Variant_Motor_4/mappedMotor_4 ==
  Vbattery : Inport
  Throttle : Inport  Port=2
  envData : Inport  Port=3
  plantData : Inport  Port=4
  3x3 Cross Product : aerolibutil/3x3 Cross Product
  Bus Selector : BusSelector  OutputSignals=V_body,CG,LLA.Altitude_m
  Bus Selector1 : BusSelector  OutputSignals=windVelocity
  Constant{1..4} (4 alike) : Constant  Value=0
  ESC_4 : Subsystem
  Motor and Propeller Coupling_4 : Subsystem
  Mux : Mux  Inputs=3
  Mux1 : Mux  Inputs=3
  Selector1 : Selector  InputPortWidth=3  IndexOptions=Index vector (dialog)  Indices=[3]  OutputSizes=1
  Selector2 : Selector  InputPortWidth=3  IndexOptions=Index vector (dialog)  Indices=[3]  OutputSizes=1
  Sum : Sum  Inputs=|+-
  Sum1 : Sum  Inputs=+-|
  Sum2 : Sum  Inputs=|++
  Terminator : Terminator
  Torque : Subsystem
  Unary Minus : UnaryMinus
  "motor2 position " : Constant  Value=LD.Propulsion.motor4.Position
  Im : Outport
  Thrust : Outport  Port=2
  Thrust_moment : Outport  Port=3
  wires:
  Constant1/1 -> Mux/2
  ESC_4/1(V_ESC) -> Motor and Propeller Coupling_4/1(Voltage)  "V_ESC"
  plantData/1 -> Bus Selector/1
  Sum1/1 -> 3x3 Cross Product/1  "arm"
  Unary Minus/1 -> Mux/3
  Constant2/1 -> Mux/1
  Bus Selector/3 -> [Altitude]  "<Altitude_m>"
  [CG] -> Sum1/2
  Bus Selector/1 -> [V_body]  "<V_body>"
  Mux/1 -> Thrust/1, 3x3 Cross Product/2  "Thrust_vector"
  Throttle/1 -> ESC_4/2(Throttle)
  Vbattery/1 -> ESC_4/1(V_battery)
  Bus Selector/2 -> [CG]  "<CG>"
  Motor and Propeller Coupling_4/1(Thrust) -> Unary Minus/1  "Thrust_scalar"
  Bus Selector1/1 -> [V_wind]  "<windVelocity>"
  [V_wind] -> Selector1/1
  "motor2 position "/1 -> Sum1/1
  envData/1 -> Bus Selector1/1
  Selector1/1 -> Sum/2
  Motor and Propeller Coupling_4/2(Power) -> Terminator/1
  [V_body] -> Selector2/1
  Selector2/1 -> Sum/1
  Motor and Propeller Coupling_4/3(Current) -> Im/1
  [Altitude] -> Motor and Propeller Coupling_4/2(Height)
  Sum/1 -> Torque/2(Vflight), Motor and Propeller Coupling_4/3(Vflight)
  Motor and Propeller Coupling_4/4(RPM) -> Torque/1(RPM)  "RPM"
  Constant4/1 -> Mux1/1
  Mux1/1 -> Sum2/2  "Torque_vector"
  Constant3/1 -> Mux1/2
  Sum2/1 -> Thrust_moment/1
  3x3 Cross Product/1 -> Sum2/1
  Torque/1(Torque) -> Mux1/3  "Torque"

== system main/LIBIS Plant/Propulsion/Variant_Motor_4/noMappedMotor_4 ==
  Vbattery : Inport
  Throttle : Inport  Port=2
  envData : Inport  Port=3
  plantData : Inport  Port=4
  3x3 Cross Product : aerolibutil/3x3 Cross Product
  Algebraic Constraint : simulink/Math Operations/Algebraic Constraint  z0=0
  Bus Selector : BusSelector  OutputSignals=V_body,CG
  Bus Selector1 : BusSelector  OutputSignals=windVelocity,AirDensity
  Constant{1..4} (4 alike) : Constant  Value=0
  ESC_4 : Subsystem
  Motor_4 : Subsystem
  Mux : Mux  Inputs=3
  Mux1 : Mux  Inputs=3
  Propeller_4 : Subsystem
  Selector1 : Selector  InputPortWidth=3  IndexOptions=Index vector (dialog)  Indices=[3]  OutputSizes=1
  Selector3 : Selector  InputPortWidth=3  IndexOptions=Index vector (dialog)  Indices=[3]  OutputSizes=1
  Sum : Sum  Inputs=|+-
  Sum1 : Sum  Inputs=+|-
  Sum2 : Sum  Inputs=|+-
  Sum3 : Sum  Inputs=++|
  Torque : Subsystem
  Unary Minus : UnaryMinus
  "motor4 position " : Constant  Value=LD.Propulsion.motor4.Position
  Im : Outport
  Thrust : Outport  Port=2
  Thrust_moment : Outport  Port=3
  wires:
  Constant1/1 -> Mux/2
  Throttle/1 -> ESC_4/2(Throttle)
  Motor_4/2(Peje) -> Sum/1  "P_available"
  Sum/1 -> Algebraic Constraint/1  "P_error"
  "motor4 position "/1 -> Sum1/1
  Algebraic Constraint/1 -> Im/1, Motor_4/2(Im)  "Im"
  Propeller_4/1(P_needed) -> Sum/2  "P_needed"
  Sum1/1 -> 3x3 Cross Product/1  "arm"
  Vbattery/1 -> ESC_4/1(V_battery)
  Mux/1 -> Thrust/1, 3x3 Cross Product/2  "Thrust_vector1"
  Constant2/1 -> Mux/1
  Propeller_4/2(Thrust) -> Unary Minus/1  "Thrust_scalar"
  Unary Minus/1 -> Mux/3
  [CG] -> Sum1/2
  ESC_4/1(V_ESC) -> Motor_4/1(V_ESC)
  plantData/1 -> Bus Selector/1
  Bus Selector/1 -> [V_body]  "<V_body>"
  Bus Selector/2 -> [CG]  "<CG>"
  [V_body] -> Selector3/1
  [V_wind] -> Selector1/1
  Selector1/1 -> Sum2/2
  Selector3/1 -> Sum2/1
  envData/1 -> Bus Selector1/1
  Bus Selector1/1 -> [V_wind]  "<windVelocity>"
  Bus Selector1/2 -> [AirDensity]  "<AirDensity>"
  [AirDensity] -> Propeller_4/3(airDensity)
  Motor_4/1(RPM) -> Torque/1(RPM), Propeller_4/1(RPM)  "RPM"
  Sum2/1 -> Torque/2(Vflight), Propeller_4/2(V_flight)
  Constant4/1 -> Mux1/1
  Constant3/1 -> Mux1/2
  Torque/1(Torque) -> Mux1/3  "Torque"
  Mux1/1 -> Sum3/1  "Torque_vector"
  3x3 Cross Product/1 -> Sum3/2
  Sum3/1 -> Thrust_moment/1

== system main/LIBIS Plant/Propulsion/Variant_Motor_5/mappedMotor_5 ==
  Vbattery : Inport
  Throttle : Inport  Port=2
  envData : Inport  Port=3
  plantData : Inport  Port=4
  3x3 Cross Product : aerolibutil/3x3 Cross Product
  Bus Selector : BusSelector  OutputSignals=V_body,CG,LLA.Altitude_m
  Bus Selector1 : BusSelector  OutputSignals=windVelocity
  Constant{1..4} (4 alike) : Constant  Value=0
  ESC_5 : Subsystem
  Motor and Propeller Coupling_5 : Subsystem
  Mux : Mux  Inputs=3
  Mux1 : Mux  Inputs=3
  Selector1 : Selector  InputPortWidth=3  IndexOptions=Index vector (dialog)  Indices=[3]  OutputSizes=1
  Selector2 : Selector  InputPortWidth=3  IndexOptions=Index vector (dialog)  Indices=[3]  OutputSizes=1
  Sum : Sum  Inputs=|+-
  Sum1 : Sum  Inputs=+-|  InputSameDT=on
  Sum2 : Sum  Inputs=|++
  Terminator : Terminator
  Torque : Subsystem
  Unary Minus : UnaryMinus
  Unary Minus1 : UnaryMinus
  "motor2 position " : Constant  Value=LD.Propulsion.motor5.Position
  Im : Outport
  Thrust : Outport  Port=2
  Thrust_moment : Outport  Port=3
  wires:
  Throttle/1 -> ESC_5/2(Throttle)
  Vbattery/1 -> ESC_5/1(V_battery)
  Selector2/1 -> Sum/1
  Selector1/1 -> Sum/2
  [CG] -> Sum1/2
  Bus Selector/3 -> [Altitude]  "<Altitude_m>"
  envData/1 -> Bus Selector1/1
  [Altitude] -> Motor and Propeller Coupling_5/2(Height)
  Bus Selector/2 -> [CG]  "<CG>"
  Motor and Propeller Coupling_5/3(Current) -> Im/1
  plantData/1 -> Bus Selector/1
  Unary Minus/1 -> Mux/3
  "motor2 position "/1 -> Sum1/1
  [V_body] -> Selector2/1
  Bus Selector1/1 -> [V_wind]  "<windVelocity>"
  [V_wind] -> Selector1/1
  Motor and Propeller Coupling_5/2(Power) -> Terminator/1
  Constant1/1 -> Mux/2
  ESC_5/1(V_ESC) -> Motor and Propeller Coupling_5/1(Voltage)  "V_ESC"
  Mux/1 -> Thrust/1, 3x3 Cross Product/2  "Thrust_vector"
  Motor and Propeller Coupling_5/1(Thrust) -> Unary Minus/1  "Thrust_scalar"
  Constant2/1 -> Mux/1
  Sum1/1 -> 3x3 Cross Product/1  "arm"
  Bus Selector/1 -> [V_body]  "<V_body>"
  Sum/1 -> Torque/2(Vflight), Motor and Propeller Coupling_5/3(Vflight)
  Motor and Propeller Coupling_5/4(RPM) -> Torque/1(RPM)  "RPM"
  Constant4/1 -> Mux1/1
  Mux1/1 -> Sum2/2  "Torque_vector"
  Constant3/1 -> Mux1/2
  Sum2/1 -> Thrust_moment/1
  3x3 Cross Product/1 -> Sum2/1
  Torque/1(Torque) -> Unary Minus1/1
  Unary Minus1/1 -> Mux1/3

== system main/LIBIS Plant/Propulsion/Variant_Motor_5/noMappedMotor_5 ==
  Vbattery : Inport
  Throttle : Inport  Port=2
  envData : Inport  Port=3
  plantData : Inport  Port=4
  3x3 Cross Product : aerolibutil/3x3 Cross Product
  Algebraic Constraint : simulink/Math Operations/Algebraic Constraint  z0=0.1
  Bus Selector : BusSelector  OutputSignals=V_body,CG
  Bus Selector1 : BusSelector  OutputSignals=windVelocity,AirDensity
  Constant{1..4} (4 alike) : Constant  Value=0
  ESC_5 : Subsystem
  Motor_5 : Subsystem
  Mux : Mux  Inputs=3
  Mux1 : Mux  Inputs=3
  Propeller_5 : Subsystem
  Selector1 : Selector  InputPortWidth=3  IndexOptions=Index vector (dialog)  Indices=[3]  OutputSizes=1
  Selector3 : Selector  InputPortWidth=3  IndexOptions=Index vector (dialog)  Indices=[3]  OutputSizes=1
  Sum : Sum  Inputs=|+-
  Sum1 : Sum  Inputs=+|-
  Sum2 : Sum  Inputs=|+-
  Sum3 : Sum  Inputs=++|
  Torque : Subsystem
  Unary Minus : UnaryMinus
  Unary Minus1 : UnaryMinus
  "motor5 position " : Constant  Value=LD.Propulsion.motor5.Position
  Im : Outport
  Thrust : Outport  Port=2
  Thrust_moment : Outport  Port=3
  wires:
  ESC_5/1(V_ESC) -> Motor_5/1(V_ESC)
  Unary Minus/1 -> Mux/3
  Propeller_5/2(Thrust) -> Unary Minus/1  "Thrust_scalar"
  Motor_5/2(Peje) -> Sum/1  "P_available"
  Throttle/1 -> ESC_5/2(Throttle)
  Propeller_5/1(P_needed) -> Sum/2  "P_needed"
  Algebraic Constraint/1 -> Im/1, Motor_5/2(Im)  "Im"
  Vbattery/1 -> ESC_5/1(V_battery)
  Sum/1 -> Algebraic Constraint/1  "P_error"
  "motor5 position "/1 -> Sum1/1
  Sum1/1 -> 3x3 Cross Product/1  "arm"
  Mux/1 -> Thrust/1, 3x3 Cross Product/2  "Thrust_vector1"
  [CG] -> Sum1/2
  Constant1/1 -> Mux/2
  Constant2/1 -> Mux/1
  plantData/1 -> Bus Selector/1
  Bus Selector/1 -> [V_body]  "<V_body>"
  Bus Selector/2 -> [CG]  "<CG>"
  [V_body] -> Selector3/1
  [V_wind] -> Selector1/1
  Selector1/1 -> Sum2/2
  Selector3/1 -> Sum2/1
  envData/1 -> Bus Selector1/1
  Bus Selector1/1 -> [V_wind]  "<windVelocity>"
  Bus Selector1/2 -> [AirDensity]  "<AirDensity>"
  [AirDensity] -> Propeller_5/3(airDensity)
  Motor_5/1(RPM) -> Torque/1(RPM), Propeller_5/1(RPM)  "RPM"
  Sum2/1 -> Torque/2(Vflight), Propeller_5/2(V_flight)
  Constant4/1 -> Mux1/1
  Constant3/1 -> Mux1/2
  Torque/1(Torque) -> Mux1/3  "Torque"
  Unary Minus1/1 -> Sum3/1
  Mux1/1 -> Unary Minus1/1  "Torque_vector"
  Sum3/1 -> Thrust_moment/1
  3x3 Cross Product/1 -> Sum3/2

== system main/LIBIS Plant/alpha_dot, beta_dot/Subsystem/calc alpha_dot ==
  q : Inport
  alpha,beta : Inport  Port=2
  Ab : Inport  Port=3
  Vw : Inport  Port=4
  Direction Cosine Matrix Body to Wind : aerolibtransform2/Direction Cosine Matrix Body to Wind
  Product1 : Product  Multiplication=Matrix(*)  SaturateOnIntegerOverflow=on  InputSameDT=on  OutDataTypeStr=Inherit: Same as first input
  Product2 : Product  Inputs=*/  SaturateOnIntegerOverflow=on  InputSameDT=on  OutDataTypeStr=Inherit: Same as first input
  Selector2 : Selector  IndexMode=Zero-based  InputPortWidth=3  IndexOptions=Index vector (dialog)  Indices=2  OutputSizes=1
  Selector3 : Selector  IndexMode=Zero-based  InputPortWidth=3  IndexOptions=Index vector (dialog)  Indices=0  OutputSizes=1
  Sum : Sum  Inputs=++|
  Transpose1 : Math  Operator=transpose  SaturateOnIntegerOverflow=on
  alpha_dot : Outport
  wires:
  Direction Cosine Matrix Body to Wind/1 -> Transpose1/1
  Transpose1/1 -> Product1/1
  Product1/1 -> Selector2/1
  Selector2/1 -> Product2/1
  Selector3/1 -> Product2/2
  Product2/1 -> Sum/2
  alpha,beta/1 -> Direction Cosine Matrix Body to Wind/1
  q/1 -> Sum/1
  Sum/1 -> alpha_dot/1
  Ab/1 -> Product1/2
  Vw/1 -> Selector3/1

== system main/Sensors/Feedthrough Sensors/IMU/Calculate DCM & Euler Angles ==
  "p q r " : Inport
  Rotation Angles to Direction Cosine Matrix : aerolibtransform2/Rotation Angles to Direction Cosine Matrix  rotationOrder=ZYX
  Selector : Selector  InputPortWidth=3  IndexOptions=Index vector (dialog)  Indices=[3 2 1]  OutputSizes=1
  phi theta psi : Integrator  InitialCondition=[initialValues.roll0 initialValues.pitch0 initialValues.yaw0]
  phidot thetadot psidot : aerolib6dofsys/DCM & Euler Angles (Euler)/phidot thetadot psidot
  DCMMeas : Outport
  EulerMeas : Outport  Port=2
  wires:
  Selector/1 -> Rotation Angles to Direction Cosine Matrix/1
  phi theta psi/1 -> EulerMeas/1, Selector/1, phidot thetadot psidot/2
  phidot thetadot psidot/1 -> phi theta psi/1
  "p q r "/1 -> phidot thetadot psidot/1
  Rotation Angles to Direction Cosine Matrix/1 -> DCMMeas/1

== system main/Sensors/Noisy Sensors/IMU/Calculate DCM & Euler Angles ==
  "p q r " : Inport
  Rotation Angles to Direction Cosine Matrix : aerolibtransform2/Rotation Angles to Direction Cosine Matrix  rotationOrder=ZYX
  Selector : Selector  InputPortWidth=3  IndexOptions=Index vector (dialog)  Indices=[3 2 1]  OutputSizes=1
  phi theta psi : Integrator  InitialCondition=[initialValues.roll0 initialValues.pitch0 initialValues.yaw0]
  phidot thetadot psidot : aerolib6dofsys/DCM & Euler Angles (Euler)/phidot thetadot psidot
  DCMMeas : Outport
  EulerMeas : Outport  Port=2
  wires:
  Selector/1 -> Rotation Angles to Direction Cosine Matrix/1
  phi theta psi/1 -> EulerMeas/1, Selector/1, phidot thetadot psidot/2
  phidot thetadot psidot/1 -> phi theta psi/1
  "p q r "/1 -> phidot thetadot psidot/1
  Rotation Angles to Direction Cosine Matrix/1 -> DCMMeas/1

== system main/LIBIS Plant/Propulsion/Variant_Motor_1/mappedMotor_1/ESC_1 ==
  V_battery : Inport  Unit=V
  Throttle : Inport  Port=2  Unit=1
  Product : Product
  Product1 : Product
  eta_ESC : Constant  Value=LD.Propulsion.ESC1.eta
  V_ESC : Outport  Unit=V
  wires:
  eta_ESC/1 -> Product/2
  V_battery/1 -> Product/1
  Product/1 -> Product1/1
  Product1/1 -> V_ESC/1
  Throttle/1 -> Product1/2
